simulink model "ControlePeO"  (R2016a)
settings: Solver=VariableStepAuto  StartTime=0.0  StopTime=0.5  RelTol=1e-3
libraries: powerlib x9, dsparch4 x2, re_lib x1, powerlib_meascontrol x1
settings Model: Creator=Jose  LastModifiedBy=Jose

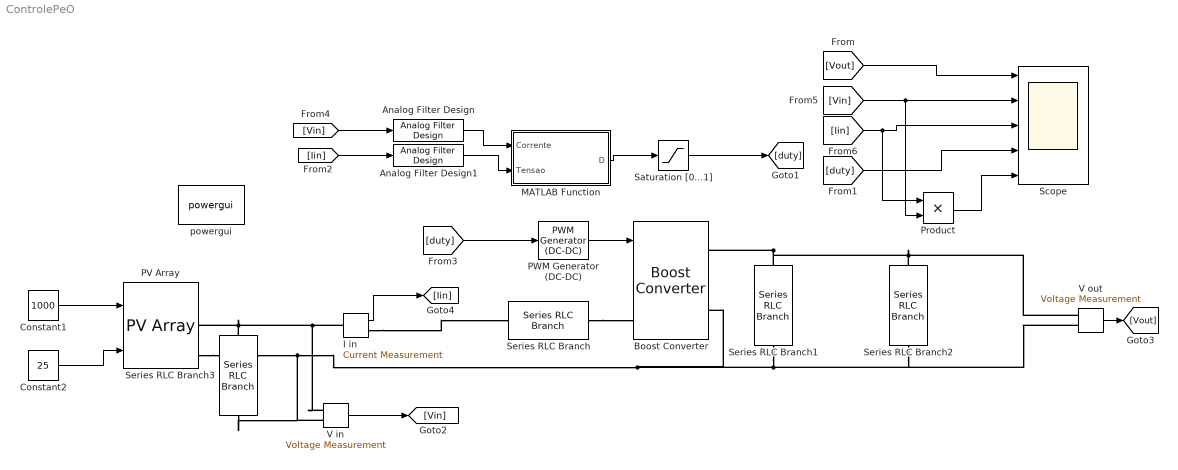
== system ControlePeO ==
  Analog Filter Design : dsparch4/Analog Filter Design  method=Butterworth  filttype=Lowpass  N=2  Wlo=2*pi*1000  Whi=80  Rp=2  Rs=40
  Analog Filter Design1 : dsparch4/Analog Filter Design  method=Butterworth  filttype=Lowpass  N=2  Wlo=2*pi*1000  Whi=80  Rp=2  Rs=40
  Boost Converter : powerlib/Power Electronics/Boost Converter  ModelType=Switching devices  Ron=0.1  Rs=1e6  Cs=inf  Vforward=[0,0]  Ron_Diode=1e-3  Rs_Diode=1e6  Cs_Diode=inf  Vf_Diode=1e-3  Rs_CurrentSource=inf
  Constant1 : Constant  Value=1000
  Constant2 : Constant  Value=25
  I in : powerlib/Measurements/Current Measurement  PhasorSimulation=off  OutputType=Complex  PSBequivalent=0
  MATLAB Function : MATLAB Function  TreatAsAtomicUnit=on
  PV Array : re_lib/Solar/PV Array  Npar=1  Nser=1  PlotType=array @ 1000 W/m2 & specified temperatures  S_vec="[ 1000  500  100 ]"  Temp_C_vec="[ 45 25  ]"  ModuleName=1Soltech 1STH-215-P  PlotWhenSelected=off  Pm=213.15  Ncell=60  Voc=36.3  Isc=7.84  Vm=29  Im=7.35  beta_Voc_pc=-0.36099  alpha_Isc_pc=0.102  beta_Voc=-0.13104  alpha_Isc=0.007997  IL=7.8649  I0=2.9259e-10  nI=0.98117  Rsh=313.3991  Rs=0.39383  BAL=off  Tc=1e-6  Tfilter=5e-5
  PWM Generator (DC-DC) : powerlib_meascontrol/Pulse & Signal Generators/PWM Generator (DC-DC)  Fsw=20000  Ts=0
  Product : Product
  Saturation [0...1] : Saturate  UpperLimit=1  LowerLimit=0
  Scope : Scope  NumInputPorts=5
  Series RLC Branch : powerlib/Elements/Series RLC Branch  LConnTagsString=__new0  RConnTagsString=__new0  BranchType=L  Resistance=1  Inductance=300e-6  SetiL0=off  InitialCurrent=0  Capacitance=1e-6  Setx0=off  InitialVoltage=0  Measurements=None
  Series RLC Branch1 : powerlib/Elements/Series RLC Branch  LConnTagsString=__new0  RConnTagsString=__new0  BranchType=C  Resistance=1  Inductance=1e-3  SetiL0=off  InitialCurrent=0  Capacitance=680e-6  Setx0=off  InitialVoltage=0  Measurements=None
  Series RLC Branch2 : powerlib/Elements/Series RLC Branch  LConnTagsString=__new0  RConnTagsString=__new0  BranchType=R  Resistance=8  Inductance=1e-3  SetiL0=off  InitialCurrent=0  Capacitance=1e-6  Setx0=off  InitialVoltage=0  Measurements=None
  Series RLC Branch3 : powerlib/Elements/Series RLC Branch  LConnTagsString=__new0  RConnTagsString=__new0  BranchType=C  Resistance=1  Inductance=1e-3  SetiL0=off  InitialCurrent=0  Capacitance=10e-6  Setx0=off  InitialVoltage=0  Measurements=None
  "V in " : powerlib/Measurements/Voltage Measurement  PhasorSimulation=off  OutputType=Complex  PSBequivalent=0
  "V out " : powerlib/Measurements/Voltage Measurement  PhasorSimulation=off  OutputType=Complex  PSBequivalent=0
  powergui : powerlib/powergui  Priority=1  SimulationMode=Continuous  SolverType=Tustin/Backward Euler (TBE)  SampleTime=50e-6  frequency=60  SPID=off  DisableSnubberDevices=off  DisableRonSwitches=off  DisableVfSwitches=off  SwTol=0  DisplayEquations=off  Interpol=off  ExternalGateDelay=off  methode=off  Ts=10  FunctionMessages=off  echomessages=off  HookPort=off  EnableUseOfTLC=off  x0status=blocks  frequencyindice=0  Pbase=100e6  ErrMax=1e-4  Iterations=50  UnitsV=kV  UnitsW=MW  buscounter=0  RestoreLinks=warning  ResistiveCurrentMeasurement=off  Frange=[0:2:500]  Ylog=off  Xlog=on  ShowGrid=off  save=off  variable=ZData  structure=0  ZoomFFT=off  StartTime=0.0  cycles=1  DisplayStyle=1  fundamental=60  FreqAxis=off  MaxFrequency=1000  frequencyindicesteady=1  RmsSteady=1  display=off
  wires:
  PWM Generator (DC-DC)/1 -> Boost Converter/1
  [Vout] -> Scope/1
  Constant2/1 -> PV Array/2
  [Iin] -> Product/1, Scope/3
  MATLAB Function/1(D) -> Saturation [0...1]/1
  Constant1/1 -> PV Array/1
  Saturation [0...1]/1 -> [duty]
  I in/1 -> [Iin]
  "V in "/1 -> [Vin]
  Analog Filter Design/1 -> MATLAB Function/1(Corrente)
  Analog Filter Design1/1 -> MATLAB Function/2(Tensao)
  [duty] -> Scope/4
  [duty] -> PWM Generator (DC-DC)/1
  "V out "/1 -> [Vout]
  [Vin] -> Analog Filter Design/1
  [Iin] -> Analog Filter Design1/1
  [Vin] -> Product/2, Scope/2
  Product/1 -> Scope/5
  connections:
  I in/LConn1 -- "V in "/LConn1 -- Series RLC Branch3/LConn1 -- PV Array/RConn1
  PV Array/RConn2 -- "V in "/LConn2 -- Series RLC Branch3/RConn1 -- Boost Converter/RConn2 -- Series RLC Branch1/RConn1 -- "V out "/LConn2 -- Series RLC Branch2/RConn1
  Series RLC Branch2/LConn1 -- Series RLC Branch1/LConn1 -- Boost Converter/RConn1 -- "V out "/LConn1
  I in/RConn1 -- Series RLC Branch/LConn1
  Series RLC Branch/RConn1 -- Boost Converter/LConn1

== matlab function ControlePeO/MATLAB Function ==
  data: Corrente input; D output; Tensao input
function D  = fcn(Corrente,Tensao)
%#codegen




Dprev = 0.1;
Vprev = 0;
Pprev = 0;


% Passo de incremento
deltaD = 0.01;

% potencia
Ppv = Tensao*Corrente;

% Algoritmo 
if (Ppv-Pprev) ~= 0
    if (Ppv-Pprev) > 0
        if (Tensao-Vprev) > 0
            D = Dprev - deltaD;
        else
            D = Dprev + deltaD;
        end
    else
        if (Tensao-Vprev) > 0
            D = Dprev + deltaD;
        else
            D = Dprev - deltaD;
        end        
    end
else
       
    D = Dprev;
end

% Atualiza valores
Dprev = D;
Vprev = Tensao;
Pprev = Corrente;
